simulink model "WheelsCanCommunication"  (R2023a)
settings: Solver=FixedStepAuto  StartTime=0.0  StopTime=5  FixedStep=1e-5  RelTol=1e-3
model workspace (MAT data in the model file):
  axltorque = 500
  breakpressure = 350
  fz = 986
  vx = 27.3
undefined symbols (not defined in the file or in its folder): canChannel
libraries: canlib x4, canmsglib x2, mspfiltlib x1, mspsensorlib x1, simulink_extras x1, autolibshared x1
(part 1 of 2)
settings Model: Creator=omert  LastModifiedBy=omert

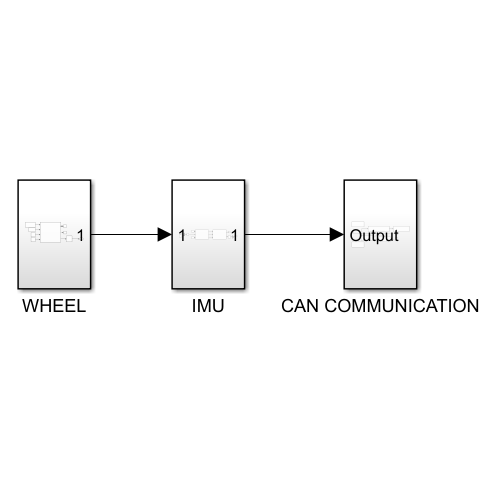
[thumbnail: Simulink's stored preview of the top-level diagram]
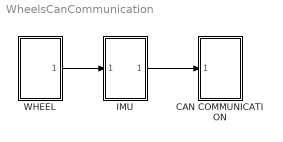
== system WheelsCanCommunication ==
  CAN COMMUNICATION : Subsystem
  IMU : Subsystem
  WHEEL : Subsystem
  wires:
  WHEEL/1(Output1) -> IMU/1(In1)
  IMU/1(Output) -> CAN COMMUNICATION/1(Output)

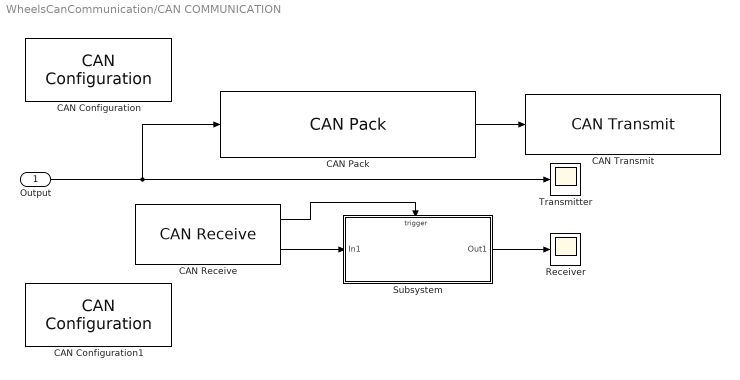
== system WheelsCanCommunication/CAN COMMUNICATION ==
  Output : Inport
  CAN Configuration : canlib/CAN Configuration  BlockHandle=4432.0002  Device=MathWorks Virtual 1 (Channel 1)  DeviceMenu=MathWorks Virtual 1 (Channel 1)  ObjConstructor=canChannel('MathWorks', 'Virtual 1', 1)  BusSpeed=500000  EnableBitParameters=off  AckMode=Normal
  CAN Configuration1 : canlib/CAN Configuration  BlockHandle=4432.0002  Device=MathWorks Virtual 1 (Channel 2)  DeviceMenu=MathWorks Virtual 1 (Channel 2)  ObjConstructor=canChannel('MathWorks', 'Virtual 1', 2)  BusSpeed=500000  EnableBitParameters=off  AckMode=Normal
  CAN Pack : canmsglib/CAN Pack  CANdbFile=C:\Users\omert\Documents\MATLAB\Examples\R2023a\vnt\GetStartedWithCANCommunicationInSimulinkExample\CANSample.dbc  MsgList=CANMessage  MsgName=CANMessage  MsgIDType=Standard (11-bit identifier)  MsgIdentifier=16  MsgLength=8  Remote=off  ApplyMinMax=off  BusOutput=off  SignalInfo={'CANSignal','0','64','LE','double','Standard','0','1','0','-1.7e+308','1.7e+308'}
      settings: LibrarySourceBlock=canlib/CAN Pack  DataFormat=CANdb specified signals
  CAN Receive : canlib/CAN Receive  BlockHandle=4442.0002  Device=MathWorks Virtual 1 (Channel 2)  DeviceMenu=MathWorks Virtual 1 (Channel 2)  ObjConstructor=canChannel('MathWorks', 'Virtual 1', 2)  EnableStandardIDsFilter=off  StdIDsCombo=Allow all  StandardIDs=0  EnableExtendedIDsFilter=off  ExtIDsCombo=Allow all  ExtendedIDs=0  SampleTime=0.01  MsgsPerTimestep=all  InternalFilterUpdateStatus=on  BusOutput=off
  CAN Transmit : canlib/CAN Transmit  BlockHandle=4445.0012  Device=MathWorks Virtual 1 (Channel 1)  DeviceMenu=MathWorks Virtual 1 (Channel 1)  ObjConstructor=canChannel('MathWorks', 'Virtual 1', 1)  EnableEventTransmit=off  EnablePeriodicTransmit=off  MessagePeriod=1.000
  Receiver : Scope
  Subsystem : Subsystem
  Transmitter : Scope
  wires:
  Output/1 -> Transmitter/1, CAN Pack/1
  CAN Pack/1 -> CAN Transmit/1
  CAN Receive/1 -> Subsystem/Trigger
  Subsystem/1(Out1) -> Receiver/1
  CAN Receive/2 -> Subsystem/1(In1)

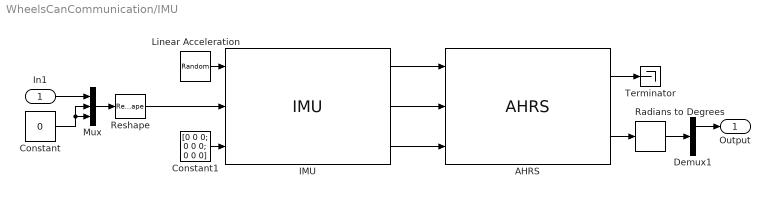
== system WheelsCanCommunication/IMU ==
  In1 : Inport
  AHRS : mspfiltlib/AHRS  DispRefFrame=NED  DecimationFactor=1  InitialProcessNoise=ahrsfilter.defaultProcessNoise  OrientationFormat=quaternion  SimulateUsing=Code generation  AccelerometerNoise=0.0001924722  GyroscopeNoise=9.1385e-5  MagnetometerNoise=0.1  GyroscopeDriftNoise=3.0462e-13  LinearAccelerationNoise=0.0096236100000000012  MagneticDisturbanceNoise=0.5  LinearAccelerationDecayFactor=0.5  MagneticDisturbanceDecayFactor=0.5  ExpectedMagneticFieldStrength=50
  Constant : Constant  Value=0
  Constant1 : Constant  Value=[0 0 0; 0 0 0; 0 0 0]
  Demux1 : Demux  Outputs=3
  IMU : mspsensorlib/IMU  DispRefFrame=NED  Temperature=25  MagneticFieldNED=[ 27.5550, -2.4169, -16.0849 ]  MagneticFieldENU=[ -2.4169, 27.5550, 16.0849 ]  SeedDouble=67  SimulateUsing=Code generation  AccelParamsMeasurementRange=19.613  AccelParamsResolution=0.0023928  AccelParamsConstantBias=[0.19 0.19 0.19]  AccelParamsAxesMisalignment=[0 0 0]  AccelParamsNoiseDensity=[0.0012356 0.0012356 0.0012356]  AccelParamsBiasInstability=[0 0 0]  AccelParamsRandomWalk=[0 0 0]  AccelParamsTemperatureBias=[0 0 0]  AccelParamsTemperatureScaleFactor=[0 0 0]  GyroParamsMeasurementRange=4.3633  GyroParamsResolution=0.0011  GyroParamsConstantBias=[0.0545 0.0545 0.0545]  GyroParamsAxesMisalignment=1.5  GyroParamsAccelerationBias=[0 0 0]  GyroParamsNoiseDensity=[0.00043633 0.00043633 0.00043633]  GyroParamsBiasInstability=[0 0 0]  GyroParamsRandomWalk=[0 0 0]  GyroParamsTemperatureBias=[0 0 0]  GyroParamsTemperatureScaleFactor=[0 0 0]  MagParamsMeasurementRange=1000  MagParamsResolution=0.1  MagParamsConstantBias=0  MagParamsAxesMisalignment=[0 0 0]  MagParamsNoiseDensity=[0.0424 0.0424 0.0424]  MagParamsBiasInstability=[0 0 0]  MagParamsRandomWalk=[0 0 0]  MagParamsTemperatureBias=[0 0 0]  MagParamsTemperatureScaleFactor=[0 0 0]
  Linear Acceleration : RandomNumber  Mean=[0 0 0]  SampleTime=0.01  VectorParams1D=off
  Mux : Mux  Inputs=3
  Radians to Degrees : simulink_extras/Transformations/Radians to Degrees
  Reshape : Reshape  OutputDimensionality=Row vector (2-D)
  Terminator : Terminator
  Output : Outport
  wires:
  Mux/1 -> Reshape/1
  IMU/1 -> AHRS/1
  Linear Acceleration/1 -> IMU/1
  IMU/2 -> AHRS/2
  IMU/3 -> AHRS/3
  AHRS/1 -> Terminator/1
  In1/1 -> Mux/1
  Constant/1 -> Mux/3, Mux/2
  Reshape/1 -> IMU/2
  Constant1/1 -> IMU/3
  AHRS/2 -> Radians to Degrees/1
  Demux1/1 -> Output/1
  Radians to Degrees/1 -> Demux1/1
